simulink library "DAQ_lib_Position"  (Simulink 8.4)
settings: Solver=ode45  StartTime=0.0  StopTime=10.0  RelTol=1e-3
undefined symbols (not defined in the file): A_lpf_velocity, ANOMALY_INIT, B1_lpf_velocity, B2_lpf_velocity, Calibration, EnableFT, EncoderAngleLimits, EncoderFiltSys, EncoderThreshold, FTCalibration, GearOffsets, IMUAngleLimits, IMUCommand, IMUThreshold, IMUTorsoOffsets, m_XR17D15x, MAX_ANOMALY, MedullaCommand, MicrostrainFiltSys, MODBUS_TIMEOUT, ResetDAQ, ResetYaw, sample_time, standard, STREAMING_TIMEOUT, TareFT, TorsoCOMOffsets, Ts, TsCAN, TsKVH, UseMicrostrainRate
libraries: xpcethercatlib x177, simulink x28, canmsglib x21, speedgoatlib x13, slrtlib x5, speedgoatlib_IO601 x5, DAQ_lib_Position x3, dspswit3 x2, dspmtrx3 x2, xpcseriallib x1, SpeedgoatModified x1
(part 4 of 6)

== system DAQ_lib_Position/DAQ Safety Stops IMU Elmo Amplifiers /DAQ/SerialInterfaces/FTCAN/CANMessageOut ==
  SelectMessage : Inport
  Merge : Merge  Inputs=9
  ReadFirmwareVersion : Subsystem
  ReadMatrixRow1 : Subsystem
  ReadMatrixRow2 : Subsystem
  ReadMatrixRow3 : Subsystem
  ReadMatrixRow4 : Subsystem
  ReadMatrixRow5 : Subsystem
  ReadMatrixRow6 : Subsystem
  ReadSGData : Subsystem
  SetActiveCalibration : Subsystem
  Switch Case : SwitchCase  CaseConditions={1,2,3,4,5,6,7,8}
  CanMessage : Outport
  wires:
  Switch Case/8 -> ReadSGData/Action
  Switch Case/1 -> SetActiveCalibration/Action
  SelectMessage/1 -> Switch Case/1
  Switch Case/2 -> ReadMatrixRow1/Action
  Switch Case/3 -> ReadMatrixRow2/Action
  Switch Case/4 -> ReadMatrixRow3/Action
  Switch Case/5 -> ReadMatrixRow4/Action
  Switch Case/6 -> ReadMatrixRow5/Action
  Switch Case/7 -> ReadMatrixRow6/Action
  Switch Case/9 -> ReadFirmwareVersion/Action
  Merge/1 -> CanMessage/1
  SetActiveCalibration/1(CanMessage) -> Merge/1
  ReadMatrixRow1/1(CanMessage) -> Merge/2
  ReadMatrixRow2/1(CanMessage) -> Merge/3
  ReadMatrixRow3/1(CanMessage) -> Merge/4
  ReadMatrixRow4/1(CanMessage) -> Merge/5
  ReadMatrixRow5/1(CanMessage) -> Merge/6
  ReadMatrixRow6/1(CanMessage) -> Merge/7
  ReadSGData/1(CanMessage) -> Merge/8
  ReadFirmwareVersion/1(CanMessage) -> Merge/9

== system DAQ_lib_Position/DAQ Safety Stops IMU Elmo Amplifiers /DAQ/SerialInterfaces/FTCAN/ComputeCalibratedTorques ==
  ZeroFT : Inport
  Cal : Inport  Port=2
  Gauge : Inport  Port=3
  ComputeCalibratedTorques : MATLAB Function  TreatAsAtomicUnit=on
  Latch : Subsystem
  Reshape : Reshape
  FT : Outport
  wires:
  Gauge/1 -> Latch/1(Gauge), ComputeCalibratedTorques/1(Gauge)
  ComputeCalibratedTorques/1(FT) -> Reshape/1
  Cal/1 -> ComputeCalibratedTorques/3(CalibrationMatrix)
  ZeroFT/1 -> Latch/Enable
  Reshape/1 -> FT/1
  Latch/1(Bias) -> ComputeCalibratedTorques/2(Bias)

== system DAQ_lib_Position/DAQ Safety Stops IMU Elmo Amplifiers /DAQ/SerialInterfaces/FTCAN/ComputeCalibratedTorques1 ==
  Tare : Inport
  Cal : Inport  Port=2
  Gauge : Inport  Port=3
  ComputeCalibratedTorques : MATLAB Function  TreatAsAtomicUnit=on
  Latch : Subsystem
  Reshape : Reshape
  FT : Outport
  wires:
  Latch/1(Bias) -> ComputeCalibratedTorques/2(Bias)
  Reshape/1 -> FT/1
  Tare/1 -> Latch/Enable
  Cal/1 -> ComputeCalibratedTorques/3(CalibrationMatrix)
  ComputeCalibratedTorques/1(FT) -> Reshape/1
  Gauge/1 -> ComputeCalibratedTorques/1(Gauge), Latch/1(Gauge)

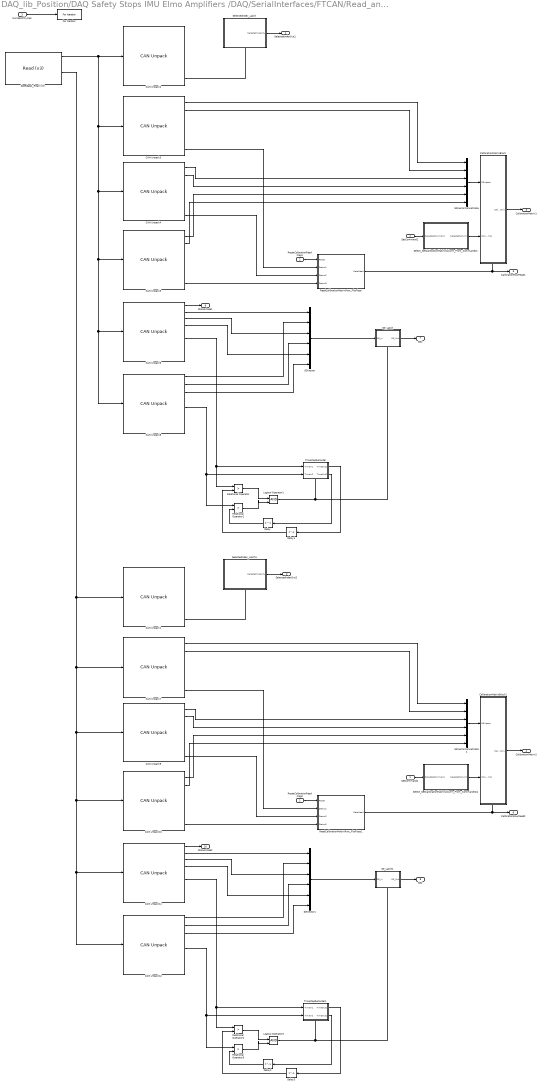
== system DAQ_lib_Position/DAQ Safety Stops IMU Elmo Amplifiers /DAQ/SerialInterfaces/FTCAN/Read_and_Process_Subsystem ==
  SetCommand1 : Inport
  ResetCalbrationReadFlag1 : Inport  Port=2
  NumberOfCycles : Inport  Port=3
  CAN Unpack1 : canmsglib/CAN Unpack  MsgList=(none)  MsgName=Read_SetActiveCalibration_Response_02  MsgIDType=Standard (11-bit identifier)  MsgIdentifier=hex2dec('206')  MsgLength=1  SignalInfo=SelectedIndex$0$8$2$2$1$0$1$0$-Inf$Inf$#  NSignals=1  IDPort=on  TimestampPort=on  ErrorPort=on  RemotePort=off  LengthPort=on  StatusPort=on  StartBits=str2num('[int32(0)]')  SignalSizes=str2num('[int32(8)]')  ByteOrders=str2num('[int32(2)]')  DataTypes=str2num('[int32(2)]')  MultiplexTypes=str2num('[int32(1)]')  MultiplexValues=str2num('[double(0)]')  Factors=str2num('[double(1)]')  Offsets=str2num('[double(0)]')  Minimums=str2num('[double(-Inf)]')  Maximums=str2num('[double(Inf)]')
  CAN Unpack10 : canmsglib/CAN Unpack  MsgList=(none)  MsgName=ReadMatrix03Response_02  MsgIDType=Standard (11-bit identifier)  MsgIdentifier=hex2dec('204')  MsgLength=8  SignalInfo=SG4$24$32$2$3$1$0$1$0$-Inf$Inf$#SG5$56$32$2$3$1$0$1$0$-Inf$Inf$#  NSignals=2  IDPort=on  TimestampPort=on  ErrorPort=on  RemotePort=off  LengthPort=on  StatusPort=on  StartBits=str2num('[int32(24);int32(56)]')  SignalSizes=str2num('[int32(32);int32(32)]')  ByteOrders=str2num('[int32(2);int32(2)]')  DataTypes=str2num('[int32(3);int32(3)]')  MultiplexTypes=str2num('[int32(1);int32(1)]')  MultiplexValues=str2num('[double(0);double(0)]')  Factors=str2num('[double(1);double(1)]')  Offsets=str2num('[double(0);double(0)]')  Minimums=str2num('[double(-Inf);double(-Inf)]')  Maximums=str2num('[double(Inf);double(Inf)]')
  CAN Unpack11 : canmsglib/CAN Unpack  MsgList=(none)  MsgName=ReadCountPerUnit_02  MsgIDType=Standard (11-bit identifier)  MsgIdentifier=hex2dec('200')  MsgLength=8  SignalInfo=StatusCode$8$16$2$2$1$0$1$0$-Inf$Inf$#SG0$24$16$2$1$1$0$1$0$-Inf$Inf$#SG2$40$16$2$1$1$0$1$0$-Inf$Inf$#SG4$56$16$2$1$1$0$1$0$-Inf$Inf$#  NSignals=4  IDPort=on  TimestampPort=on  ErrorPort=on  RemotePort=off  LengthPort=on  StatusPort=on  StartBits=str2num('[int32(8);int32(24);int32(40);int32(56)]')  SignalSizes=str2num('[int32(16);int32(16);int32(16);int32(16)]')  ByteOrders=str2num('[int32(2);int32(2);int32(2);int32(2)]')  DataTypes=str2num('[int32(2);int32(1);int32(1);int32(1)]')  MultiplexTypes=str2num('[int32(1);int32(1);int32(1);int32(1)]')  MultiplexValues=str2num('[double(0);double(0);double(0);double(0)]')  Factors=str2num('[double(1);double(1);double(1);double(1)]')  Offsets=str2num('[double(0);double(0);double(0);double(0)]')  Minimums=str2num('[double(-Inf);double(-Inf);double(-Inf);double(-Inf)]')  Maximums=str2num('[double(Inf);double(Inf);double(Inf);double(Inf)]')
  CAN Unpack12 : canmsglib/CAN Unpack  MsgList=(none)  MsgName=ReadCountPerUnit_02  MsgIDType=Standard (11-bit identifier)  MsgIdentifier=hex2dec('201')  MsgLength=6  SignalInfo=SG1$8$16$2$1$1$0$1$0$-Inf$Inf$#SG3$24$16$2$1$1$0$1$0$-Inf$Inf$#SG5$40$16$2$1$1$0$1$0$-Inf$Inf$#  NSignals=3  IDPort=on  TimestampPort=on  ErrorPort=on  RemotePort=off  LengthPort=on  StatusPort=on  StartBits=str2num('[int32(8);int32(24);int32(40)]')  SignalSizes=str2num('[int32(16);int32(16);int32(16)]')  ByteOrders=str2num('[int32(2);int32(2);int32(2)]')  DataTypes=str2num('[int32(1);int32(1);int32(1)]')  MultiplexTypes=str2num('[int32(1);int32(1);int32(1)]')  MultiplexValues=str2num('[double(0);double(0);double(0)]')  Factors=str2num('[double(1);double(1);double(1)]')  Offsets=str2num('[double(0);double(0);double(0)]')  Minimums=str2num('[double(-Inf);double(-Inf);double(-Inf)]')  Maximums=str2num('[double(Inf);double(Inf);double(Inf)]')
  CAN Unpack2 : canmsglib/CAN Unpack  MsgList=(none)  MsgName=Read_SetActiveCalibration_Response_01  MsgIDType=Standard (11-bit identifier)  MsgIdentifier=hex2dec('206')  MsgLength=1  SignalInfo=SelectedIndex$0$8$2$2$1$0$1$0$-Inf$Inf$#  NSignals=1  IDPort=on  TimestampPort=on  ErrorPort=on  RemotePort=off  LengthPort=on  StatusPort=on  StartBits=str2num('[int32(0)]')  SignalSizes=str2num('[int32(8)]')  ByteOrders=str2num('[int32(2)]')  DataTypes=str2num('[int32(2)]')  MultiplexTypes=str2num('[int32(1)]')  MultiplexValues=str2num('[double(0)]')  Factors=str2num('[double(1)]')  Offsets=str2num('[double(0)]')  Minimums=str2num('[double(-Inf)]')  Maximums=str2num('[double(Inf)]')
  CAN Unpack3 : canmsglib/CAN Unpack  MsgList=(none)  MsgName=ReadMatrix01Response_01  MsgIDType=Standard (11-bit identifier)  MsgIdentifier=hex2dec('202')  MsgLength=8  SignalInfo=SG0$24$32$2$3$1$0$1$0$-Inf$Inf$#SG1$56$32$2$3$1$0$1$0$-Inf$Inf$#  NSignals=2  IDPort=on  TimestampPort=on  ErrorPort=on  RemotePort=off  LengthPort=on  StatusPort=on  StartBits=str2num('[int32(24);int32(56)]')  SignalSizes=str2num('[int32(32);int32(32)]')  ByteOrders=str2num('[int32(2);int32(2)]')  DataTypes=str2num('[int32(3);int32(3)]')  MultiplexTypes=str2num('[int32(1);int32(1)]')  MultiplexValues=str2num('[double(0);double(0)]')  Factors=str2num('[double(1);double(1)]')  Offsets=str2num('[double(0);double(0)]')  Minimums=str2num('[double(-Inf);double(-Inf)]')  Maximums=str2num('[double(Inf);double(Inf)]')
  CAN Unpack4 : canmsglib/CAN Unpack  MsgList=(none)  MsgName=ReadMatrix02Response_01  MsgIDType=Standard (11-bit identifier)  MsgIdentifier=hex2dec('203')  MsgLength=8  SignalInfo=SG2$24$32$2$3$1$0$1$0$-Inf$Inf$#SG3$56$32$2$3$1$0$1$0$-Inf$Inf$#  NSignals=2  IDPort=on  TimestampPort=on  ErrorPort=on  RemotePort=off  LengthPort=on  StatusPort=on  StartBits=str2num('[int32(24);int32(56)]')  SignalSizes=str2num('[int32(32);int32(32)]')  ByteOrders=str2num('[int32(2);int32(2)]')  DataTypes=str2num('[int32(3);int32(3)]')  MultiplexTypes=str2num('[int32(1);int32(1)]')  MultiplexValues=str2num('[double(0);double(0)]')  Factors=str2num('[double(1);double(1)]')  Offsets=str2num('[double(0);double(0)]')  Minimums=str2num('[double(-Inf);double(-Inf)]')  Maximums=str2num('[double(Inf);double(Inf)]')
  CAN Unpack5 : canmsglib/CAN Unpack  MsgList=(none)  MsgName=ReadMatrix03Response_01  MsgIDType=Standard (11-bit identifier)  MsgIdentifier=hex2dec('204')  MsgLength=8  SignalInfo=SG4$24$32$2$3$1$0$1$0$-Inf$Inf$#SG5$56$32$2$3$1$0$1$0$-Inf$Inf$#  NSignals=2  IDPort=on  TimestampPort=on  ErrorPort=on  RemotePort=off  LengthPort=on  StatusPort=on  StartBits=str2num('[int32(24);int32(56)]')  SignalSizes=str2num('[int32(32);int32(32)]')  ByteOrders=str2num('[int32(2);int32(2)]')  DataTypes=str2num('[int32(3);int32(3)]')  MultiplexTypes=str2num('[int32(1);int32(1)]')  MultiplexValues=str2num('[double(0);double(0)]')  Factors=str2num('[double(1);double(1)]')  Offsets=str2num('[double(0);double(0)]')  Minimums=str2num('[double(-Inf);double(-Inf)]')  Maximums=str2num('[double(Inf);double(Inf)]')
  CAN Unpack6 : canmsglib/CAN Unpack  MsgList=(none)  MsgName=ReadCountPerUnit_01  MsgIDType=Standard (11-bit identifier)  MsgIdentifier=hex2dec('200')  MsgLength=8  SignalInfo=StatusCode$8$16$2$2$1$0$1$0$-Inf$Inf$#SG0$24$16$2$1$1$0$1$0$-Inf$Inf$#SG2$40$16$2$1$1$0$1$0$-Inf$Inf$#SG4$56$16$2$1$1$0$1$0$-Inf$Inf$#  NSignals=4  IDPort=on  TimestampPort=on  ErrorPort=on  RemotePort=off  LengthPort=on  StatusPort=on  StartBits=str2num('[int32(8);int32(24);int32(40);int32(56)]')  SignalSizes=str2num('[int32(16);int32(16);int32(16);int32(16)]')  ByteOrders=str2num('[int32(2);int32(2);int32(2);int32(2)]')  DataTypes=str2num('[int32(2);int32(1);int32(1);int32(1)]')  MultiplexTypes=str2num('[int32(1);int32(1);int32(1);int32(1)]')  MultiplexValues=str2num('[double(0);double(0);double(0);double(0)]')  Factors=str2num('[double(1);double(1);double(1);double(1)]')  Offsets=str2num('[double(0);double(0);double(0);double(0)]')  Minimums=str2num('[double(-Inf);double(-Inf);double(-Inf);double(-Inf)]')  Maximums=str2num('[double(Inf);double(Inf);double(Inf);double(Inf)]')
  CAN Unpack7 : canmsglib/CAN Unpack  MsgList=(none)  MsgName=ReadMatrix01Response_02  MsgIDType=Standard (11-bit identifier)  MsgIdentifier=hex2dec('202')  MsgLength=8  SignalInfo=SG0$24$32$2$3$1$0$1$0$-Inf$Inf$#SG1$56$32$2$3$1$0$1$0$-Inf$Inf$#  NSignals=2  IDPort=on  TimestampPort=on  ErrorPort=on  RemotePort=off  LengthPort=on  StatusPort=on  StartBits=str2num('[int32(24);int32(56)]')  SignalSizes=str2num('[int32(32);int32(32)]')  ByteOrders=str2num('[int32(2);int32(2)]')  DataTypes=str2num('[int32(3);int32(3)]')  MultiplexTypes=str2num('[int32(1);int32(1)]')  MultiplexValues=str2num('[double(0);double(0)]')  Factors=str2num('[double(1);double(1)]')  Offsets=str2num('[double(0);double(0)]')  Minimums=str2num('[double(-Inf);double(-Inf)]')  Maximums=str2num('[double(Inf);double(Inf)]')
  CAN Unpack8 : canmsglib/CAN Unpack  MsgList=(none)  MsgName=ReadCountPerUnit_01  MsgIDType=Standard (11-bit identifier)  MsgIdentifier=hex2dec('201')  MsgLength=6  SignalInfo=SG1$8$16$2$1$1$0$1$0$-Inf$Inf$#SG3$24$16$2$1$1$0$1$0$-Inf$Inf$#SG5$40$16$2$1$1$0$1$0$-Inf$Inf$#  NSignals=3  IDPort=on  TimestampPort=on  ErrorPort=on  RemotePort=off  LengthPort=on  StatusPort=on  StartBits=str2num('[int32(8);int32(24);int32(40)]')  SignalSizes=str2num('[int32(16);int32(16);int32(16)]')  ByteOrders=str2num('[int32(2);int32(2);int32(2)]')  DataTypes=str2num('[int32(1);int32(1);int32(1)]')  MultiplexTypes=str2num('[int32(1);int32(1);int32(1)]')  MultiplexValues=str2num('[double(0);double(0);double(0)]')  Factors=str2num('[double(1);double(1);double(1)]')  Offsets=str2num('[double(0);double(0);double(0)]')  Minimums=str2num('[double(-Inf);double(-Inf);double(-Inf)]')  Maximums=str2num('[double(Inf);double(Inf);double(Inf)]')
  CAN Unpack9 : canmsglib/CAN Unpack  MsgList=(none)  MsgName=ReadMatrix02Response_02  MsgIDType=Standard (11-bit identifier)  MsgIdentifier=hex2dec('203')  MsgLength=8  SignalInfo=SG2$24$32$2$3$1$0$1$0$-Inf$Inf$#SG3$56$32$2$3$1$0$1$0$-Inf$Inf$#  NSignals=2  IDPort=on  TimestampPort=on  ErrorPort=on  RemotePort=off  LengthPort=on  StatusPort=on  StartBits=str2num('[int32(24);int32(56)]')  SignalSizes=str2num('[int32(32);int32(32)]')  ByteOrders=str2num('[int32(2);int32(2)]')  DataTypes=str2num('[int32(3);int32(3)]')  MultiplexTypes=str2num('[int32(1);int32(1)]')  MultiplexValues=str2num('[double(0);double(0)]')  Factors=str2num('[double(1);double(1)]')  Offsets=str2num('[double(0);double(0)]')  Minimums=str2num('[double(-Inf);double(-Inf)]')  Maximums=str2num('[double(Inf);double(Inf)]')
  CalibrationMatrixBlock : Subsystem
  CalibrationMatrixBlock1 : Subsystem
  Delay{,1..3} (4 alike) : Delay  DelayLength=1  InitialCondition=0
  For Iterator : ForIterator  IterationSource=external  IterationLimit=2  ShowIterationPort=off
  Logical Operator1 : Logic  IconShape=distinctive  AllPortsSameDT=off  OutDataTypeStr=boolean
  Logical Operator3 : Logic  IconShape=distinctive  AllPortsSameDT=off  OutDataTypeStr=boolean
  ReadCalibrationMatrixRow_FlipFlops : Subsystem
  ReadCalibrationMatrixRow_FlipFlops1 : Subsystem
  Relational Operator{,1..3} (4 alike) : RelationalOperator  Operator=>  OutDataTypeStr=boolean
  ResetCalbrationReadFlag2 : InportShadow  Port=2
  SGVector : Concatenate  NumInputs=6
  SGVector1 : Concatenate  NumInputs=6
  SGVectorConcatinate : Concatenate  NumInputs=6
  SGVectorConcatinate1 : Concatenate  NumInputs=6
  SG_Latch : Subsystem
  SG_Latch1 : Subsystem
  Select_SetCalibrationMatrixColumn_From_CommandNo : Subsystem
  Select_SetCalibrationMatrixColumn_From_CommandNo1 : Subsystem
  SelectedIndex_Latch : Subsystem
  SelectedIndex_Latch1 : Subsystem
  SetCommand2 : InportShadow
  Speedgoat_Read (v3) : speedgoatlib_IO601/Read (v3)  id=1  outputFormat=Vector of CAN_MESSAGE  port1=on  port2=on  depth1=1  depth2=1  sampletime=-1  pciSlot=-1
  TimestapRecorder : Subsystem
  TimestapRecorder1 : Subsystem
  SelectedIndexOut1 : Outport
  SelectedIndexOut2 : Outport  Port=2
  CalibrationMatrix1 : Outport  Port=3
  CalibrationMatrix2 : Outport  Port=4
  CalibrationRowRead1 : Outport  Port=5
  CalibrationRowRead2 : Outport  Port=6
  SG1 : Outport  Port=7
  SG2 : Outport  Port=8
  StatusCode1 : Outport  Port=9
  StatusCode2 : Outport  Port=10
  wires:
  CAN Unpack3/1 -> SGVectorConcatinate/1
  CAN Unpack3/2 -> SGVectorConcatinate/2
  CAN Unpack4/1 -> SGVectorConcatinate/3
  CAN Unpack4/2 -> SGVectorConcatinate/4
  CAN Unpack5/1 -> SGVectorConcatinate/5
  CAN Unpack5/2 -> SGVectorConcatinate/6
  CAN Unpack2/6 -> SelectedIndex_Latch/Enable
  CAN Unpack4/7 -> ReadCalibrationMatrixRow_FlipFlops/3(Status2)
  SGVectorConcatinate/1 -> CalibrationMatrixBlock/1(SGVector)
  SetCommand1/1 -> Select_SetCalibrationMatrixColumn_From_CommandNo/1(SelectedCommand)
  Select_SetCalibrationMatrixColumn_From_CommandNo/1(SelectedColumn) -> CalibrationMatrixBlock/2(ColumnNo)
  CalibrationMatrixBlock/1(CalibrationMatrix) -> CalibrationMatrix1/1
  CAN Unpack3/7 -> ReadCalibrationMatrixRow_FlipFlops/2(Status1)
  CAN Unpack5/7 -> ReadCalibrationMatrixRow_FlipFlops/4(Status3)
  ResetCalbrationReadFlag1/1 -> ReadCalibrationMatrixRow_FlipFlops/1(Reset)
  CAN Unpack6/2 -> SGVector/1
  CAN Unpack8/1 -> SGVector/2
  CAN Unpack6/3 -> SGVector/3
  CAN Unpack8/2 -> SGVector/4
  CAN Unpack6/4 -> SGVector/5
  CAN Unpack8/3 -> SGVector/6
  SG_Latch/1(SG_Out) -> SG1/1
  SGVector/1 -> SG_Latch/1(SG_In)
  CAN Unpack8/5 -> TimestapRecorder/2(TimeIn2), Relational Operator1/1
  Relational Operator/1 -> Logical Operator1/1
  Relational Operator1/1 -> Logical Operator1/2
  Logical Operator1/1 -> SG_Latch/Enable, TimestapRecorder/Enable
  CAN Unpack6/6 -> TimestapRecorder/1(TimeIn1), Relational Operator/1
  TimestapRecorder/2(TimeOut2) -> Delay/1
  TimestapRecorder/1(TimeOut1) -> Delay1/1
  Delay/1 -> Relational Operator1/2
  Delay1/1 -> Relational Operator/2
  CAN Unpack7/1 -> SGVectorConcatinate1/1
  CAN Unpack7/2 -> SGVectorConcatinate1/2
  CAN Unpack9/1 -> SGVectorConcatinate1/3
  CAN Unpack9/2 -> SGVectorConcatinate1/4
  CAN Unpack10/1 -> SGVectorConcatinate1/5
  CAN Unpack10/2 -> SGVectorConcatinate1/6
  CAN Unpack1/6 -> SelectedIndex_Latch1/Enable
  CAN Unpack9/7 -> ReadCalibrationMatrixRow_FlipFlops1/3(Status2)
  SGVectorConcatinate1/1 -> CalibrationMatrixBlock1/1(SGVector)
  Select_SetCalibrationMatrixColumn_From_CommandNo1/1(SelectedColumn) -> CalibrationMatrixBlock1/2(ColumnNo)
  CalibrationMatrixBlock1/1(CalibrationMatrix) -> CalibrationMatrix2/1
  CAN Unpack7/7 -> ReadCalibrationMatrixRow_FlipFlops1/2(Status1)
  CAN Unpack10/7 -> ReadCalibrationMatrixRow_FlipFlops1/4(Status3)
  CAN Unpack11/2 -> SGVector1/1
  CAN Unpack12/1 -> SGVector1/2
  CAN Unpack11/3 -> SGVector1/3
  CAN Unpack12/2 -> SGVector1/4
  CAN Unpack11/4 -> SGVector1/5
  CAN Unpack12/3 -> SGVector1/6
  SG_Latch1/1(SG_Out) -> SG2/1
  SGVector1/1 -> SG_Latch1/1(SG_In)
  CAN Unpack12/5 -> TimestapRecorder1/2(TimeIn2), Relational Operator3/1
  Relational Operator2/1 -> Logical Operator3/1
  Relational Operator3/1 -> Logical Operator3/2
  Logical Operator3/1 -> SG_Latch1/Enable, TimestapRecorder1/Enable
  CAN Unpack11/6 -> TimestapRecorder1/1(TimeIn1), Relational Operator2/1
  TimestapRecorder1/2(TimeOut2) -> Delay2/1
  TimestapRecorder1/1(TimeOut1) -> Delay3/1
  Delay2/1 -> Relational Operator3/2
  Delay3/1 -> Relational Operator2/2
  ResetCalbrationReadFlag2/1 -> ReadCalibrationMatrixRow_FlipFlops1/1(Reset)
  SetCommand2/1 -> Select_SetCalibrationMatrixColumn_From_CommandNo1/1(SelectedCommand)
  ReadCalibrationMatrixRow_FlipFlops/1(DataRead) -> CalibrationRowRead1/1, CalibrationMatrixBlock/Enable
  ReadCalibrationMatrixRow_FlipFlops1/1(DataRead) -> CalibrationRowRead2/1, CalibrationMatrixBlock1/Enable
  SelectedIndex_Latch/1(SelectedIndexOut) -> SelectedIndexOut1/1
  SelectedIndex_Latch1/1(SelectedIndexOut) -> SelectedIndexOut2/1
  CAN Unpack6/1 -> StatusCode1/1
  CAN Unpack11/1 -> StatusCode2/1
  Speedgoat_Read (v3)/1 -> CAN Unpack8/1, CAN Unpack6/1, CAN Unpack5/1, CAN Unpack4/1, CAN Unpack3/1, CAN Unpack2/1
  NumberOfCycles/1 -> For Iterator/1
  Speedgoat_Read (v3)/3 -> CAN Unpack12/1, CAN Unpack11/1, CAN Unpack10/1, CAN Unpack9/1, CAN Unpack7/1, CAN Unpack1/1

== system DAQ_lib_Position/DAQ Safety Stops IMU Elmo Amplifiers /DAQ/SerialInterfaces/FTInterface/ATI Serial NoInt ==
  TX1 : Inport
  TX2 : Inport  Port=2
  Board Setup : speedgoatlib/IO503/Speedgoat IO503 Internal blocks/Board Setup  irqnum=9  slot=slot
  Constant : Constant  OutDataTypeStr=Inherit: Inherit via back propagation  SampleTime=-1
  Constant1 : Constant  OutDataTypeStr=Inherit: Inherit via back propagation  SampleTime=-1
  Count : Selector  IndexMode=Zero-based  Indices=0
  Count1 : Selector  IndexMode=Zero-based  Indices=0
  Read HW FIFO : speedgoatlib/IO503/Speedgoat IO503 Internal blocks/Read HW FIFO  port=1  flush=off  slot=slot
  Read HW FIFO1 : speedgoatlib/IO503/Speedgoat IO503 Internal blocks/Read HW FIFO  port=2  flush=off  slot=slot
  Setup 2 : speedgoatlib/IO503/Speedgoat IO503 Internal blocks/Setup  port=2  transceiver=RS485 half-duplex  standard=on  baudrate=1382400  bauddivisor=1  mode8x=16x (standard)  prescale=off  width=8  nstop=1  parity=Even  rlevel=almost full (56)  ctsmode=none  xonoff=none  xon=17  xoff=19  rs485mode=on  rs485delay=0  slot=slot
  "Setup1 " : speedgoatlib/IO503/Speedgoat IO503 Internal blocks/Setup  port=1  transceiver=RS485 half-duplex  standard=on  baudrate=1382400  bauddivisor=1  mode8x=16x (standard)  prescale=off  width=8  nstop=1  parity=Even  rlevel=almost full (56)  ctsmode=none  xonoff=none  xon=17  xoff=19  rs485mode=on  rs485delay=0  slot=slot
  Write HW FIFO : speedgoatlib/IO503/Speedgoat IO503 Internal blocks/Write HW FIFO  port=1  slot=slot
  Write HW FIFO1 : speedgoatlib/IO503/Speedgoat IO503 Internal blocks/Write HW FIFO  port=2  slot=slot
  RX1 : Outport  SourceOfInitialOutputValue=Input signal
  RX2 : Outport  Port=2  SourceOfInitialOutputValue=Input signal
  wires:
  Read HW FIFO/1 -> RX1/1
  Constant/1 -> Read HW FIFO/1
  Read HW FIFO1/1 -> RX2/1
  Constant1/1 -> Read HW FIFO1/1
  Count/1 -> Write HW FIFO/2
  Count1/1 -> Write HW FIFO1/2
  TX1/1 -> Count/1, Write HW FIFO/1
  TX2/1 -> Count1/1, Write HW FIFO1/1

== system DAQ_lib_Position/DAQ Safety Stops IMU Elmo Amplifiers /DAQ/SerialInterfaces/FTInterface/Subsystem ==
  CalibrationSet : Inport  Partition=off
  Tare : Inport  Port=2  Partition=off
  Reset : Inport  Port=3  Partition=off
  SerialIn : Inport  Port=4  Partition=on  PartitionDimension=1  PartitionWidth=65
  ComputeCalibratedTorques : Subsystem
  FTStateMachine : Stateflow chart  TreatAsAtomicUnit=on
  For Each : ForEach  DisableCoverage=on  IndexMode=One-based
  FTStatus : Outport  ConcatenationDimension=1
  FT : Outport  Port=2  ConcatenationDimension=1
  FTInterfaceStatus : Outport  Port=3  ConcatenationDimension=1
  FTSetupStatus : Outport  Port=4  ConcatenationDimension=1
  CalibrationSerial : Outport  Port=5  ConcatenationDimension=1
  SerialOut : Outport  Port=6  ConcatenationDimension=1
  wires:
  SerialIn/1 -> FTStateMachine/3(SerialIn)
  FTStateMachine/4(FTInterfaceStatus) -> FTInterfaceStatus/1
  FTStateMachine/6(SerialOut) -> SerialOut/1
  CalibrationSet/1 -> FTStateMachine/1(CalibrationSet)
  FTStateMachine/5(FTSetupStatus) -> FTSetupStatus/1
  ComputeCalibratedTorques/1(FT) -> FT/1
  FTStateMachine/3(Calibration) -> ComputeCalibratedTorques/2(Cal)
  FTStateMachine/1(GaugeStatus) -> FTStatus/1
  Tare/1 -> ComputeCalibratedTorques/3(Tare)
  Reset/1 -> FTStateMachine/2(Reset)
  FTStateMachine/2(Gauge) -> ComputeCalibratedTorques/1(Gauge)

== system DAQ_lib_Position/DAQ Safety Stops IMU Elmo Amplifiers /DAQ/SerialInterfaces/KVH/Send Receive1 ==
  Board Setup : speedgoatlib/IO503/Speedgoat IO503 Internal blocks/Board Setup  irqnum=9  slot=slot
  Constant : Constant
  Read HW FIFO : speedgoatlib/IO503/Speedgoat IO503 Internal blocks/Read HW FIFO  port=1  flush=on  slot=slot
  Setup3 : speedgoatlib/IO503/Speedgoat IO503 Internal blocks/Setup  port=3  transceiver=RS422  standard=on  baudrate=921600  bauddivisor=1  mode8x=16x (standard)  prescale=off  width=8  nstop=1  parity=None  rlevel=half full (32)  ctsmode=none  xonoff=none  xon=17  xoff=19  rs485mode=off  rs485delay=0  slot=slot
  Rx3 : Outport
  wires:
  Read HW FIFO/1 -> Rx3/1
  Constant/1 -> Read HW FIFO/1

== system DAQ_lib_Position/DAQ Safety Stops IMU Elmo Amplifiers /DAQ/SerialInterfaces/KVH/Subsystem ==
  Board Setup : speedgoatlib/IO503/Speedgoat IO503 Internal blocks/Board Setup  irqnum=5  slot=slot
  Constant : Constant  OutDataTypeStr=uint32  SampleTime=-1
  FIFO write 1 : xpcseriallib/FIFO write   size=256  inputtype=count+32 bit uint  present=off  sampletime=-1  id=IO503: KVH Interface
  Read HW FIFO : speedgoatlib/IO503/Speedgoat IO503 Internal blocks/Read HW FIFO  port=3  flush=on  slot=slot
  Setup3 : speedgoatlib/IO503/Speedgoat IO503 Internal blocks/Setup  port=3  transceiver=RS422  standard=on  baudrate=921600  bauddivisor=1  mode8x=16x (standard)  prescale=off  width=8  nstop=1  parity=None  rlevel=almost full (56)  ctsmode=none  xonoff=none  xon=17  xoff=19  rs485mode=off  rs485delay=0  slot=slot
  SerialData : Outport
  wires:
  Constant/1 -> Read HW FIFO/1
  Read HW FIFO/1 -> FIFO write 1/1
  FIFO write 1/1 -> SerialData/1

== system DAQ_lib_Position/DAQ Safety Stops IMU Elmo Amplifiers /DAQ/SerialInterfaces/KVH/UpdateOrientation ==
  FIFO : Inport
  Reset : Inport  Port=2
  Assignment : Assignment  IndexMode=Zero-based  IndexOptions=Index vector (port)
  Assignment1 : Assignment  IndexMode=Zero-based  IndexOptions=Index vector (port)
  Constant : Constant  Value=[0; 0]
  Constant1 : Constant  Value=0  OutDataTypeStr=uint8
  Constant2 : Constant  Value=[0; 0]
  Data Type Conversion : DataTypeConversion  OutDataTypeStr=double
  Data Type Conversion1 : DataTypeConversion  OutDataTypeStr=uint8  RndMeth=Simplest
  Data Type Conversion2 : DataTypeConversion  OutDataTypeStr=double
  Data Type Conversion3 : DataTypeConversion  OutDataTypeStr=double
  EstimateOrientation : MATLAB Function  TreatAsAtomicUnit=on
  "FIFO bin read " : SpeedgoatModified/FIFO Read Binary Multiple  header={char([254, 129, 255, 85])}  lengths=36  hold=Zero output if no new data  enable=off  maxsize=36  outputtype=count+32 bit uint  sampletime=-1
  For Iterator : ForIterator  IterationLimit=2  IndexMode=Zero-based
  MATLAB Function : MATLAB Function  TreatAsAtomicUnit=on
  Selector : Selector  IndexMode=Zero-based  InputPortWidth=37  Indices=1:36
  Selector1 : Selector  IndexMode=Zero-based  InputPortWidth=37  Indices=0
  Switch : Switch  Criteria=u2 > Threshold
  Unit Delay : UnitDelay  InitialCondition=[0; 0; 0]  SampleTime=-1
  Unit Delay1 : UnitDelay  InitialCondition=zeros(3,3)  SampleTime=-1
  Unit Delay2 : UnitDelay  InitialCondition=[0; 0; 0]  SampleTime=-1
  Unit Delay3 : UnitDelay  SampleTime=-1
  Rk : Outport  InitialOutput=zeros(3,3)
  wk : Outport  Port=2  InitialOutput=zeros(3,1)
  DeltaAngle : Outport  Port=3  InitialOutput=zeros(3,1)
  Acceleration : Outport  Port=4  InitialOutput=zeros(3,1)
  Status : Outport  Port=5  InitialOutput=0
  Sequence : Outport  Port=6  InitialOutput=[0; 0]
  Temperature : Outport  Port=7  InitialOutput=0
  Valid : Outport  Port=8  InitialOutput=0
  PacketSize : Outport  Port=9  InitialOutput=0
  wires:
  MATLAB Function/2(Acceleration) -> Acceleration/1, EstimateOrientation/2(Acceleration)
  MATLAB Function/1(Rotation) -> DeltaAngle/1, EstimateOrientation/1(DeltaAngle)
  MATLAB Function/3(Status) -> Data Type Conversion1/1
  MATLAB Function/5(Temperature) -> Temperature/1
  EstimateOrientation/3(Ak) -> Unit Delay/1
  Unit Delay/1 -> EstimateOrientation/8(Akm1)
  EstimateOrientation/1(Rk) -> Rk/1, Unit Delay1/1
  Unit Delay1/1 -> EstimateOrientation/6(Rkm1)
  [Reset] -> EstimateOrientation/5(Reset)
  Switch/1 -> EstimateOrientation/3(Status)
  MATLAB Function/6(Valid) -> Switch/2, Data Type Conversion/1
  EstimateOrientation/4(Seqk) -> Unit Delay3/1
  Unit Delay3/1 -> EstimateOrientation/9(Seqkm1)
  Reset/1 -> [Reset]
  FIFO/1 -> "FIFO bin read "/1
  EstimateOrientation/2(wk) -> wk/1, Unit Delay2/1
  Unit Delay2/1 -> EstimateOrientation/7(wkm1)
  "FIFO bin read "/1 -> Selector1/1, Selector/1
  MATLAB Function/4(Sequence) -> EstimateOrientation/4(Sequence), Assignment/2
  Assignment/1 -> Sequence/1
  Constant/1 -> Assignment/1
  Selector/1 -> MATLAB Function/1(P)
  Data Type Conversion/1 -> Valid/1
  Data Type Conversion1/1 -> Data Type Conversion2/1, Switch/1
  Constant1/1 -> Switch/3
  Data Type Conversion2/1 -> Status/1
  Selector1/1 -> Data Type Conversion3/1
  Constant2/1 -> Assignment1/1
  For Iterator/1 -> Assignment1/3, Assignment/3
  Assignment1/1 -> PacketSize/1
  Data Type Conversion3/1 -> Assignment1/2

== system DAQ_lib_Position/DAQ Safety Stops IMU Elmo Amplifiers /DAQ/EtherCATNetwork/EncoderFilters/CheckAndFilterEncoder/OSU_filter ==
  q : Inport
  Gain1 : Gain  Gain=1/sample_time
  difference : simulink/Discrete/Difference  ICPrevInput=0  InputProcessing=Columns as channels (frame based)  OutMin=[]  OutMax=[]  OutDataType=fixdt(1, 16)  OutScaling=2^-10  DoSatur=off
  two_pole_filter : DiscreteTransferFcn  Numerator=[A_lpf_velocity 0 0]  Denominator=[1 B1_lpf_velocity B2_lpf_velocity]  SampleTime=sample_time
  dq : Outport
  wires:
  Gain1/1 -> two_pole_filter/1
  two_pole_filter/1 -> dq/1
  q/1 -> difference/1
  difference/1 -> Gain1/1

== system DAQ_lib_Position/DAQ Safety Stops IMU Elmo Amplifiers /DAQ/EtherCATNetwork/EtherCATRobotMicrostrain/LegElmo_1L/EtherCATSubsystem ==
  Control Word : Inport
  Mode of Operation : Inport  Port=2
  Target Position : Inport  Port=3
  Target Velocity : Inport  Port=4
  Target Torque : Inport  Port=5
  EtherCAT PDO Receive : xpcethercatlib/EtherCAT PDO Receive  Priority=2  sig_name=Drive 1 (Elmo Drive).Inputs.Status word  sig_offset=592  sig_type=uint16  type_size=16  sig_dim=1  device_id=0  sample_time=0.000500
  EtherCAT PDO Receive1 : xpcethercatlib/EtherCAT PDO Receive  Priority=2  sig_name=Drive 1 (Elmo Drive).Inputs.Mode of operation display  sig_offset=608  sig_type=int8  type_size=8  sig_dim=1  device_id=0  sample_time=0.000500
  EtherCAT PDO Receive2 : xpcethercatlib/EtherCAT PDO Receive  Priority=2  sig_name=Drive 1 (Elmo Drive).Inputs.Torque actual value  sig_offset=688  sig_type=int16  type_size=16  sig_dim=1  device_id=0  sample_time=0.000500
  EtherCAT PDO Receive3 : xpcethercatlib/EtherCAT PDO Receive  Priority=2  sig_name=Drive 1 (Elmo Drive).Inputs.Actual position [counts]  sig_offset=624  sig_type=int32  type_size=32  sig_dim=1  device_id=0  sample_time=0.000500
  EtherCAT PDO Receive4 : xpcethercatlib/EtherCAT PDO Receive  Priority=2  sig_name=Drive 1 (Elmo Drive).Inputs.Velocity actual value  sig_offset=656  sig_type=int32  type_size=32  sig_dim=1  device_id=0  sample_time=0.000500
  EtherCAT PDO Transmit : xpcethercatlib/EtherCAT PDO Transmit   Priority=3  sig_name=Drive 1 (Elmo Drive).Outputs.Control word  sig_offset=592  sig_type=uint16  type_size=16  sig_dim=1  device_id=0  sample_time=0.000500
  EtherCAT PDO Transmit1 : xpcethercatlib/EtherCAT PDO Transmit   Priority=3  sig_name=Drive 1 (Elmo Drive).Outputs.Mode of operation  sig_offset=608  sig_type=int8  type_size=8  sig_dim=1  device_id=0  sample_time=0.000500
  EtherCAT PDO Transmit2 : xpcethercatlib/EtherCAT PDO Transmit   Priority=3  sig_name=Drive 1 (Elmo Drive).Outputs.Target Position  sig_offset=640  sig_type=int32  type_size=32  sig_dim=1  device_id=0  sample_time=0.000500
  EtherCAT PDO Transmit3 : xpcethercatlib/EtherCAT PDO Transmit   Priority=3  sig_name=Drive 1 (Elmo Drive).Outputs.Target Velocity  sig_offset=672  sig_type=int32  type_size=32  sig_dim=1  device_id=0  sample_time=0.000500
  EtherCAT PDO Transmit4 : xpcethercatlib/EtherCAT PDO Transmit   Priority=3  sig_name=Drive 1 (Elmo Drive).Outputs.Target Torque  sig_offset=624  sig_type=int16  type_size=16  sig_dim=1  device_id=0  sample_time=0.000500
  Status Word : Outport
  Mode of Operation Display : Outport  Port=2
  Actual Position : Outport  Port=3
  Actual Velocity : Outport  Port=4
  Actual Torque : Outport  Port=5
  wires:
  EtherCAT PDO Receive/1 -> Status Word/1
  EtherCAT PDO Receive1/1 -> Mode of Operation Display/1
  Mode of Operation/1 -> EtherCAT PDO Transmit1/1
  EtherCAT PDO Receive3/1 -> Actual Position/1
  EtherCAT PDO Receive4/1 -> Actual Velocity/1
  Target Position/1 -> EtherCAT PDO Transmit2/1
  EtherCAT PDO Receive2/1 -> Actual Torque/1
  Control Word/1 -> EtherCAT PDO Transmit/1
  Target Velocity/1 -> EtherCAT PDO Transmit3/1
  Target Torque/1 -> EtherCAT PDO Transmit4/1

== system DAQ_lib_Position/DAQ Safety Stops IMU Elmo Amplifiers /DAQ/EtherCATNetwork/EtherCATRobotMicrostrain/LegElmo_1L/Subsystem1 ==
  ControlWordIndex : Inport
  EnableControlWord : Subsystem
  FaultReset : Subsystem
  Merge : Merge  Inputs=4
  NothingControlWord : Subsystem
  ShutdownControlWord : Subsystem
  Switch Case : SwitchCase  CaseConditions={1,2,3}
  ControlWord : Outport
  wires:
  NothingControlWord/1(ControlWord) -> Merge/4
  Merge/1 -> ControlWord/1
  Switch Case/1 -> ShutdownControlWord/Action
  ShutdownControlWord/1(ControlWord) -> Merge/1
  Switch Case/4 -> NothingControlWord/Action
  Switch Case/2 -> EnableControlWord/Action
  ControlWordIndex/1 -> Switch Case/1
  EnableControlWord/1(ControlWord) -> Merge/2
  Switch Case/3 -> FaultReset/Action
  FaultReset/1(ControlWord) -> Merge/3

== system DAQ_lib_Position/DAQ Safety Stops IMU Elmo Amplifiers /DAQ/EtherCATNetwork/EtherCATRobotMicrostrain/LegElmo_1L/Subsystem10 ==
  ActualValue : Inport
  MaxRatedCurrent : Inport  Port=2
  Data Type Conversion6 : DataTypeConversion  OutDataTypeStr=int16
  Fcn : Fcn  Expr=u(1)*1000/u(2)
  Vector Concatenate : Concatenate
  ScaledValue : Outport
  wires:
  ActualValue/1 -> Vector Concatenate/1
  Vector Concatenate/1 -> Fcn/1
  MaxRatedCurrent/1 -> Vector Concatenate/2
  Data Type Conversion6/1 -> ScaledValue/1
  Fcn/1 -> Data Type Conversion6/1

== system DAQ_lib_Position/DAQ Safety Stops IMU Elmo Amplifiers /DAQ/EtherCATNetwork/EtherCATRobotMicrostrain/LegElmo_1L/Subsystem2 ==
  StatusWord : Inport
  Bitwise Operator : simulink/Logic and Bit Operations/Bitwise Operator  logicop=AND  UseBitMask=on  BitMask=bin2dec('0000000001001111')  BitMaskRealWorld=Stored Integer
  Compare To Constant : simulink/Logic and Bit Operations/Compare To Constant  relop===  const=bin2dec('0000000001000000')  OutDataTypeStr=boolean
  SwitchOnDisabledMode : Outport
  wires:
  StatusWord/1 -> Bitwise Operator/1
  Compare To Constant/1 -> SwitchOnDisabledMode/1
  Bitwise Operator/1 -> Compare To Constant/1

== system DAQ_lib_Position/DAQ Safety Stops IMU Elmo Amplifiers /DAQ/EtherCATNetwork/EtherCATRobotMicrostrain/LegElmo_1L/Subsystem3 ==
  StatusWord : Inport
  Bitwise Operator : simulink/Logic and Bit Operations/Bitwise Operator  logicop=AND  UseBitMask=on  BitMask=bin2dec('0000000001101111')  BitMaskRealWorld=Stored Integer
  Compare To Constant : simulink/Logic and Bit Operations/Compare To Constant  relop===  const=bin2dec('0000000000100111')  OutDataTypeStr=boolean
  EnabledMode : Outport
  wires:
  StatusWord/1 -> Bitwise Operator/1
  Compare To Constant/1 -> EnabledMode/1
  Bitwise Operator/1 -> Compare To Constant/1

== system DAQ_lib_Position/DAQ Safety Stops IMU Elmo Amplifiers /DAQ/EtherCATNetwork/EtherCATRobotMicrostrain/LegElmo_1L/Subsystem4 ==
  StatusWord : Inport
  Bitwise Operator : simulink/Logic and Bit Operations/Bitwise Operator  logicop=AND  UseBitMask=on  BitMask=bin2dec('0000000001101111')  BitMaskRealWorld=Stored Integer
  Compare To Constant : simulink/Logic and Bit Operations/Compare To Constant  relop===  const=bin2dec('0000000000100001')  OutDataTypeStr=boolean
  ReadyToSwitchOnMode : Outport
  wires:
  StatusWord/1 -> Bitwise Operator/1
  Compare To Constant/1 -> ReadyToSwitchOnMode/1
  Bitwise Operator/1 -> Compare To Constant/1

== system DAQ_lib_Position/DAQ Safety Stops IMU Elmo Amplifiers /DAQ/EtherCATNetwork/EtherCATRobotMicrostrain/LegElmo_1L/Subsystem5 ==
  StatusWord : Inport
  Bitwise Operator : simulink/Logic and Bit Operations/Bitwise Operator  logicop=AND  UseBitMask=on  BitMask=bin2dec('0000000000001000')  BitMaskRealWorld=Stored Integer
  Compare To Constant : simulink/Logic and Bit Operations/Compare To Constant  relop===  const=bin2dec('0000000000001000')  OutDataTypeStr=boolean
  FaultMode : Outport
  wires:
  StatusWord/1 -> Bitwise Operator/1
  Compare To Constant/1 -> FaultMode/1
  Bitwise Operator/1 -> Compare To Constant/1

== system DAQ_lib_Position/DAQ Safety Stops IMU Elmo Amplifiers /DAQ/EtherCATNetwork/EtherCATRobotMicrostrain/LegElmo_1L/Subsystem6 ==
  ScaledValue : Inport
  MaxRatedCurrent : Inport  Port=2
  Fcn : Fcn  Expr=u(1)*u(2)/1000
  Vector Concatenate : Concatenate
  ActualValue : Outport
  wires:
  ScaledValue/1 -> Vector Concatenate/1
  Vector Concatenate/1 -> Fcn/1
  MaxRatedCurrent/1 -> Vector Concatenate/2
  Fcn/1 -> ActualValue/1

== system DAQ_lib_Position/DAQ Safety Stops IMU Elmo Amplifiers /DAQ/SerialInterfaces/FTCAN/CANMessageOut/ReadFirmwareVersion ==
  Action Port : ActionPort
  CAN Pack : canmsglib/CAN Pack  MsgList=(none)  MsgName=ReadFirmwareVersion  MsgIDType=Standard (11-bit identifier)  MsgIdentifier=hex2dec('20F')  MsgLength=0  NSignals=0  StartBits=0  SignalSizes=0  ByteOrders=0  DataTypes=0  MultiplexTypes=0  MultiplexValues=0  Factors=0  Offsets=0  Minimums=0  Maximums=0  Remote=off
      settings: DataFormat=manually specified signals
  Constant : Constant  Value=0  SampleTime=TsCAN
  CanMessage : Outport
  wires:
  CAN Pack/1 -> CanMessage/1
  Constant/1 -> CAN Pack/1

== system DAQ_lib_Position/DAQ Safety Stops IMU Elmo Amplifiers /DAQ/SerialInterfaces/FTCAN/CANMessageOut/ReadMatrixRow1 ==
  Action Port : ActionPort
  CAN Pack : canmsglib/CAN Pack  MsgList=(none)  MsgName=ReadMatrix  MsgIDType=Standard (11-bit identifier)  MsgIdentifier=hex2dec('202')  MsgLength=1  SignalInfo=AxisRow$0$8$1$2$1$0$1$0$-Inf$Inf$#  NSignals=1  StartBits=str2num('[int32(0)]')  SignalSizes=str2num('[int32(8)]')  ByteOrders=str2num('[int32(1)]')  DataTypes=str2num('[int32(2)]')  MultiplexTypes=str2num('[int32(1)]')  MultiplexValues=str2num('[double(0)]')  Factors=str2num('[double(1)]')  Offsets=str2num('[double(0)]')  Minimums=str2num('[double(-Inf)]')  Maximums=str2num('[double(Inf)]')  Remote=off
      settings: DataFormat=manually specified signals
  Constant : Constant  Value=0  SampleTime=TsCAN
  CanMessage : Outport
  wires:
  CAN Pack/1 -> CanMessage/1
  Constant/1 -> CAN Pack/1

== system DAQ_lib_Position/DAQ Safety Stops IMU Elmo Amplifiers /DAQ/SerialInterfaces/FTCAN/CANMessageOut/ReadMatrixRow2 ==
  Action Port : ActionPort
  CAN Pack : canmsglib/CAN Pack  MsgList=(none)  MsgName=ReadMatrix  MsgIDType=Standard (11-bit identifier)  MsgIdentifier=hex2dec('202')  MsgLength=1  SignalInfo=AxisRow$0$8$1$2$1$0$1$0$-Inf$Inf$#  NSignals=1  StartBits=str2num('[int32(0)]')  SignalSizes=str2num('[int32(8)]')  ByteOrders=str2num('[int32(1)]')  DataTypes=str2num('[int32(2)]')  MultiplexTypes=str2num('[int32(1)]')  MultiplexValues=str2num('[double(0)]')  Factors=str2num('[double(1)]')  Offsets=str2num('[double(0)]')  Minimums=str2num('[double(-Inf)]')  Maximums=str2num('[double(Inf)]')  Remote=off
      settings: DataFormat=manually specified signals
  Constant : Constant  SampleTime=TsCAN
  CanMessage : Outport
  wires:
  CAN Pack/1 -> CanMessage/1
  Constant/1 -> CAN Pack/1

== system DAQ_lib_Position/DAQ Safety Stops IMU Elmo Amplifiers /DAQ/SerialInterfaces/FTCAN/CANMessageOut/ReadMatrixRow3 ==
  Action Port : ActionPort
  CAN Pack : canmsglib/CAN Pack  MsgList=(none)  MsgName=ReadMatrix  MsgIDType=Standard (11-bit identifier)  MsgIdentifier=hex2dec('202')  MsgLength=1  SignalInfo=AxisRow$0$8$1$2$1$0$1$0$-Inf$Inf$#  NSignals=1  StartBits=str2num('[int32(0)]')  SignalSizes=str2num('[int32(8)]')  ByteOrders=str2num('[int32(1)]')  DataTypes=str2num('[int32(2)]')  MultiplexTypes=str2num('[int32(1)]')  MultiplexValues=str2num('[double(0)]')  Factors=str2num('[double(1)]')  Offsets=str2num('[double(0)]')  Minimums=str2num('[double(-Inf)]')  Maximums=str2num('[double(Inf)]')  Remote=off
      settings: DataFormat=manually specified signals
  Constant : Constant  Value=2  SampleTime=TsCAN
  CanMessage : Outport
  wires:
  CAN Pack/1 -> CanMessage/1
  Constant/1 -> CAN Pack/1

== system DAQ_lib_Position/DAQ Safety Stops IMU Elmo Amplifiers /DAQ/SerialInterfaces/FTCAN/CANMessageOut/ReadMatrixRow4 ==
  Action Port : ActionPort
  CAN Pack : canmsglib/CAN Pack  MsgList=(none)  MsgName=ReadMatrix  MsgIDType=Standard (11-bit identifier)  MsgIdentifier=hex2dec('202')  MsgLength=1  SignalInfo=AxisRow$0$8$1$2$1$0$1$0$-Inf$Inf$#  NSignals=1  StartBits=str2num('[int32(0)]')  SignalSizes=str2num('[int32(8)]')  ByteOrders=str2num('[int32(1)]')  DataTypes=str2num('[int32(2)]')  MultiplexTypes=str2num('[int32(1)]')  MultiplexValues=str2num('[double(0)]')  Factors=str2num('[double(1)]')  Offsets=str2num('[double(0)]')  Minimums=str2num('[double(-Inf)]')  Maximums=str2num('[double(Inf)]')  Remote=off
      settings: DataFormat=manually specified signals
  Constant : Constant  Value=3  SampleTime=TsCAN
  CanMessage : Outport
  wires:
  CAN Pack/1 -> CanMessage/1
  Constant/1 -> CAN Pack/1

== system DAQ_lib_Position/DAQ Safety Stops IMU Elmo Amplifiers /DAQ/SerialInterfaces/FTCAN/CANMessageOut/ReadMatrixRow5 ==
  Action Port : ActionPort
  CAN Pack : canmsglib/CAN Pack  MsgList=(none)  MsgName=ReadMatrix  MsgIDType=Standard (11-bit identifier)  MsgIdentifier=hex2dec('202')  MsgLength=1  SignalInfo=AxisRow$0$8$1$2$1$0$1$0$-Inf$Inf$#  NSignals=1  StartBits=str2num('[int32(0)]')  SignalSizes=str2num('[int32(8)]')  ByteOrders=str2num('[int32(1)]')  DataTypes=str2num('[int32(2)]')  MultiplexTypes=str2num('[int32(1)]')  MultiplexValues=str2num('[double(0)]')  Factors=str2num('[double(1)]')  Offsets=str2num('[double(0)]')  Minimums=str2num('[double(-Inf)]')  Maximums=str2num('[double(Inf)]')  Remote=off
      settings: DataFormat=manually specified signals
  Constant : Constant  Value=4  SampleTime=TsCAN
  CanMessage : Outport
  wires:
  CAN Pack/1 -> CanMessage/1
  Constant/1 -> CAN Pack/1

== system DAQ_lib_Position/DAQ Safety Stops IMU Elmo Amplifiers /DAQ/SerialInterfaces/FTCAN/CANMessageOut/ReadMatrixRow6 ==
  Action Port : ActionPort
  CAN Pack : canmsglib/CAN Pack  MsgList=(none)  MsgName=ReadMatrix  MsgIDType=Standard (11-bit identifier)  MsgIdentifier=hex2dec('202')  MsgLength=1  SignalInfo=AxisRow$0$8$1$2$1$0$1$0$-Inf$Inf$#  NSignals=1  StartBits=str2num('[int32(0)]')  SignalSizes=str2num('[int32(8)]')  ByteOrders=str2num('[int32(1)]')  DataTypes=str2num('[int32(2)]')  MultiplexTypes=str2num('[int32(1)]')  MultiplexValues=str2num('[double(0)]')  Factors=str2num('[double(1)]')  Offsets=str2num('[double(0)]')  Minimums=str2num('[double(-Inf)]')  Maximums=str2num('[double(Inf)]')  Remote=off
      settings: DataFormat=manually specified signals
  Constant : Constant  Value=5  SampleTime=TsCAN
  CanMessage : Outport
  wires:
  CAN Pack/1 -> CanMessage/1
  Constant/1 -> CAN Pack/1

== system DAQ_lib_Position/DAQ Safety Stops IMU Elmo Amplifiers /DAQ/SerialInterfaces/FTCAN/CANMessageOut/ReadSGData ==
  Action Port : ActionPort
  CAN Pack : canmsglib/CAN Pack  MsgList=(none)  MsgName=ReadFTSerialNumber  MsgIDType=Standard (11-bit identifier)  MsgIdentifier=hex2dec('200')  MsgLength=0  NSignals=0  StartBits=0  SignalSizes=0  ByteOrders=0  DataTypes=0  MultiplexTypes=0  MultiplexValues=0  Factors=0  Offsets=0  Minimums=0  Maximums=0  Remote=off
      settings: DataFormat=manually specified signals
  Constant : Constant  Value=0  SampleTime=TsCAN
  CanMessage : Outport
  wires:
  CAN Pack/1 -> CanMessage/1
  Constant/1 -> CAN Pack/1

== system DAQ_lib_Position/DAQ Safety Stops IMU Elmo Amplifiers /DAQ/SerialInterfaces/FTCAN/CANMessageOut/SetActiveCalibration ==
  Action Port : ActionPort
  CAN Pack : canmsglib/CAN Pack  MsgList=(none)  MsgName=SetActiveCommand  MsgIDType=Standard (11-bit identifier)  MsgIdentifier=hex2dec('206')  MsgLength=1  SignalInfo=CalibrationIndex$0$8$1$2$1$0$1$0$-Inf$Inf$#  NSignals=1  StartBits=str2num('[int32(0)]')  SignalSizes=str2num('[int32(8)]')  ByteOrders=str2num('[int32(1)]')  DataTypes=str2num('[int32(2)]')  MultiplexTypes=str2num('[int32(1)]')  MultiplexValues=str2num('[double(0)]')  Factors=str2num('[double(1)]')  Offsets=str2num('[double(0)]')  Minimums=str2num('[double(-Inf)]')  Maximums=str2num('[double(Inf)]')  Remote=off
      settings: DataFormat=manually specified signals
  Constant : Constant  Value=0  SampleTime=TsCAN
  CanMessage : Outport
  wires:
  CAN Pack/1 -> CanMessage/1
  Constant/1 -> CAN Pack/1

== system DAQ_lib_Position/DAQ Safety Stops IMU Elmo Amplifiers /DAQ/SerialInterfaces/FTCAN/ComputeCalibratedTorques/Latch ==
  Gauge : Inport
  Tare : EnablePort
  Bias : Outport  InitialOutput=zeros(6,1,'uint16')
  wires:
  Gauge/1 -> Bias/1

== system DAQ_lib_Position/DAQ Safety Stops IMU Elmo Amplifiers /DAQ/SerialInterfaces/FTCAN/ComputeCalibratedTorques1/Latch ==
  Gauge : Inport
  Tare : EnablePort
  Bias : Outport  InitialOutput=zeros(6,1,'uint16')
  wires:
  Gauge/1 -> Bias/1

== system DAQ_lib_Position/DAQ Safety Stops IMU Elmo Amplifiers /DAQ/SerialInterfaces/FTCAN/Read_and_Process_Subsystem/CalibrationMatrixBlock ==
  SGVector : Inport
  ColumnNo : Inport  Port=2
  Enable : EnablePort
  Compare To Constant : simulink/Logic and Bit Operations/Compare To Constant  relop===  const=1  OutDataTypeStr=boolean
  Compare To Constant1 : simulink/Logic and Bit Operations/Compare To Constant  relop===  const=2  OutDataTypeStr=boolean
  Compare To Constant2 : simulink/Logic and Bit Operations/Compare To Constant  relop===  const=3  OutDataTypeStr=boolean
  Compare To Constant3 : simulink/Logic and Bit Operations/Compare To Constant  relop===  const=4  OutDataTypeStr=boolean
  Compare To Constant4 : simulink/Logic and Bit Operations/Compare To Constant  relop===  const=5  OutDataTypeStr=boolean
  Compare To Constant5 : simulink/Logic and Bit Operations/Compare To Constant  relop===  const=6  OutDataTypeStr=boolean
  Fx : Subsystem
  Fy : Subsystem
  Fz : Subsystem
  Matrix Concatenate : Concatenate  NumInputs=6  Mode=Multidimensional array
  Transpose : dspmtrx3/Transpose  Hermitian=off  overflowFlag=off
  Tx : Subsystem
  Ty : Subsystem
  Tz : Subsystem
  CalibrationMatrix : Outport
  wires:
  Compare To Constant/1 -> Fx/Enable
  Compare To Constant1/1 -> Fy/Enable
  Compare To Constant2/1 -> Fz/Enable
  Compare To Constant3/1 -> Tx/Enable
  Compare To Constant4/1 -> Ty/Enable
  Compare To Constant5/1 -> Tz/Enable
  ColumnNo/1 -> Compare To Constant1/1, Compare To Constant5/1, Compare To Constant4/1, Compare To Constant3/1, Compare To Constant2/1, Compare To Constant/1
  Fx/1(Out) -> Matrix Concatenate/1
  Fy/1(Out) -> Matrix Concatenate/2
  Fz/1(Out) -> Matrix Concatenate/3
  Tx/1(Out) -> Matrix Concatenate/4
  Ty/1(Out) -> Matrix Concatenate/5
  Tz/1(Out) -> Matrix Concatenate/6
  Matrix Concatenate/1 -> CalibrationMatrix/1
  SGVector/1 -> Transpose/1
  Transpose/1 -> Tz/1(In), Ty/1(In), Tx/1(In), Fz/1(In), Fy/1(In), Fx/1(In)

== system DAQ_lib_Position/DAQ Safety Stops IMU Elmo Amplifiers /DAQ/SerialInterfaces/FTCAN/Read_and_Process_Subsystem/CalibrationMatrixBlock1 ==
  SGVector : Inport
  ColumnNo : Inport  Port=2
  Enable : EnablePort
  Compare To Constant : simulink/Logic and Bit Operations/Compare To Constant  relop===  const=1  OutDataTypeStr=boolean
  Compare To Constant1 : simulink/Logic and Bit Operations/Compare To Constant  relop===  const=2  OutDataTypeStr=boolean
  Compare To Constant2 : simulink/Logic and Bit Operations/Compare To Constant  relop===  const=3  OutDataTypeStr=boolean
  Compare To Constant3 : simulink/Logic and Bit Operations/Compare To Constant  relop===  const=4  OutDataTypeStr=boolean
  Compare To Constant4 : simulink/Logic and Bit Operations/Compare To Constant  relop===  const=5  OutDataTypeStr=boolean
  Compare To Constant5 : simulink/Logic and Bit Operations/Compare To Constant  relop===  const=6  OutDataTypeStr=boolean
  Fx : Subsystem
  Fy : Subsystem
  Fz : Subsystem
  Matrix Concatenate : Concatenate  NumInputs=6  Mode=Multidimensional array
  Transpose : dspmtrx3/Transpose  Hermitian=off  overflowFlag=off
  Tx : Subsystem
  Ty : Subsystem
  Tz : Subsystem
  CalibrationMatrix : Outport
  wires:
  Compare To Constant/1 -> Fx/Enable
  Compare To Constant1/1 -> Fy/Enable
  Compare To Constant2/1 -> Fz/Enable
  Compare To Constant3/1 -> Tx/Enable
  Compare To Constant4/1 -> Ty/Enable
  Compare To Constant5/1 -> Tz/Enable
  ColumnNo/1 -> Compare To Constant1/1, Compare To Constant5/1, Compare To Constant4/1, Compare To Constant3/1, Compare To Constant2/1, Compare To Constant/1
  Fx/1(Out) -> Matrix Concatenate/1
  Fy/1(Out) -> Matrix Concatenate/2
  Fz/1(Out) -> Matrix Concatenate/3
  Tx/1(Out) -> Matrix Concatenate/4
  Ty/1(Out) -> Matrix Concatenate/5
  Tz/1(Out) -> Matrix Concatenate/6
  Matrix Concatenate/1 -> CalibrationMatrix/1
  SGVector/1 -> Transpose/1
  Transpose/1 -> Tz/1(In), Ty/1(In), Tx/1(In), Fz/1(In), Fy/1(In), Fx/1(In)

== system DAQ_lib_Position/DAQ Safety Stops IMU Elmo Amplifiers /DAQ/SerialInterfaces/FTCAN/Read_and_Process_Subsystem/ReadCalibrationMatrixRow_FlipFlops ==
  Reset : Inport
  Status1 : Inport  Port=2
  Status2 : Inport  Port=3
  Status3 : Inport  Port=4
  Logical Operator : Logic  Inputs=3  IconShape=distinctive  AllPortsSameDT=off  OutDataTypeStr=boolean
  Logical Operator1 : Logic  Operator=OR  IconShape=distinctive  AllPortsSameDT=off  OutDataTypeStr=boolean
  Logical Operator2 : Logic  Operator=OR  IconShape=distinctive  AllPortsSameDT=off  OutDataTypeStr=boolean
  Logical Operator3 : Logic  Operator=OR  IconShape=distinctive  AllPortsSameDT=off  OutDataTypeStr=boolean
  Subsystem : Subsystem
  Subsystem1 : Subsystem
  Subsystem2 : Subsystem
  DataRead : Outport
  wires:
  Status1/1 -> Logical Operator1/2, Subsystem/1(Status)
  Reset/1 -> Subsystem2/2(Reset), Logical Operator3/1, Subsystem1/2(Reset), Logical Operator2/1, Subsystem/2(Reset), Logical Operator1/1
  Status2/1 -> Logical Operator2/2, Subsystem1/1(Status)
  Status3/1 -> Logical Operator3/2, Subsystem2/1(Status)
  Subsystem2/1(StatusLatched) -> Logical Operator/3
  Subsystem1/1(StatusLatched) -> Logical Operator/2
  Subsystem/1(StatusLatched) -> Logical Operator/1
  Logical Operator1/1 -> Subsystem/Enable
  Logical Operator2/1 -> Subsystem1/Enable
  Logical Operator3/1 -> Subsystem2/Enable
  Logical Operator/1 -> DataRead/1
